simulink model "Local_webcam_test"  (Simulink 7.8)
settings: Solver=ode45  StartTime=0.0  StopTime=10.0  RelTol=1e-3
undefined symbols (not defined in the file): jet, none, videoinput
libraries: visionsinks x2, imaqlib x1
settings Model: Creator=wildcat  LastModifiedBy=wildcat
settings DebuggingCC: FcnCallInpInsideContextMsg=Use local settings  StrictBusMsg=Warning
settings SFSimCC: SimParseCustomCode=off

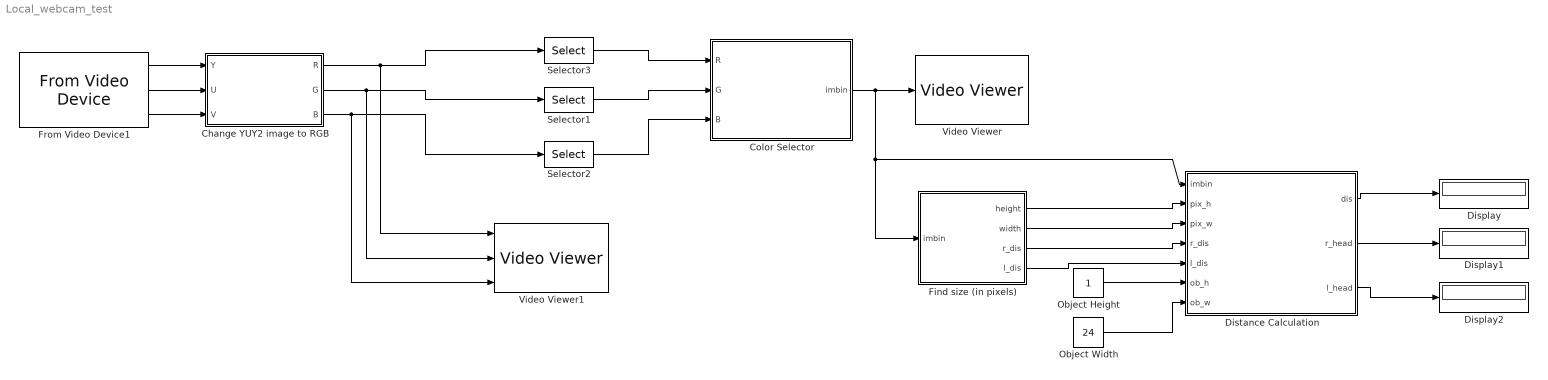
== system Local_webcam_test ==
  Change YUY2 image to RGB : MATLAB Function  TreatAsAtomicUnit=on
  Color Selector : MATLAB Function  TreatAsAtomicUnit=on
  Display : Display
  Display1 : Display
  Display2 : Display
  Distance Calculation : MATLAB Function  TreatAsAtomicUnit=on
  Find size (in pixels) : MATLAB Function  TreatAsAtomicUnit=on
  From Video Device1 : imaqlib/From Video Device  DeviceMenu=winvideo 1 (Microsoft LifeCam HD-3000)  Device=winvideo 1 (Microsoft LifeCam HD-3000)  ObjConstructor=videoinput('winvideo', 1)  VideoFormatMenu=YUY2_640x480  VideoFormat=YUY2_640x480  VideoSource=input1  ROIPosition=[0 0 480 640]  EnableHWTrigger=off  TriggerConfiguration=none/none  SampleTime=1/30  OutputPortsMode=Separate color signals  DataType=uint8  CanDoHWTrigger=no  ReturnedColorSpace=YCbCr  BlockHandle=2599.0059  ROIWidth=640  ROIHeight=480  ROIColumn=0  ROIRow=0  EngXMLPath=C:\Program Files\MatlabR2011b\toolbox\imaq\imaq\private  DevXMLPath=C:\Program Files\MatlabR2011b\toolbox\imaq\imaqadaptors\win64  EngLibPath=C:\Program Files\MatlabR2011b\toolbox\imaq\imaqblks\imaqmex\win64
  Object Height : Constant
  Object Width : Constant  Value=24
  Selector1 : Selector  NumberOfDimensions=2  InputPortWidth=3  IndexOptions=Starting index (dialog),Starting index (dialog)  Indices=70,1  OutputSizes=340,640
  Selector2 : Selector  NumberOfDimensions=2  InputPortWidth=3  IndexOptions=Starting index (dialog),Starting index (dialog)  Indices=70,1  OutputSizes=340,640
  Selector3 : Selector  NumberOfDimensions=2  InputPortWidth=3  IndexOptions=Starting index (dialog),Starting index (dialog)  Indices=70,1  OutputSizes=340,640
  Video Viewer : visionsinks/Video Viewer  inputType=Obsolete7b  imagePorts=One multidimensional signal  useColorMap=off  colormapValue=jet(256)  specRange=off  minInputVal=0  maxInputVal=255  FigPos=[840 554 410 300]  AxisZoom=on  trueSizedOnce=off  OpenAtMdlStart=on
  Video Viewer1 : visionsinks/Video Viewer  inputType=Obsolete7b  imagePorts=Separate color signals  useColorMap=off  colormapValue=jet(256)  specRange=off  minInputVal=0  maxInputVal=255  FigPos=[314 546 410 300]  AxisZoom=on  trueSizedOnce=off  OpenAtMdlStart=on
  wires:
  Color Selector/1(imbin) -> Find size (in pixels)/1(imbin), Distance Calculation/1(imbin), Video Viewer/1
  Find size (in pixels)/1(height) -> Distance Calculation/2(pix_h)
  Find size (in pixels)/2(width) -> Distance Calculation/3(pix_w)
  Object Height/1 -> Distance Calculation/6(ob_h)
  Object Width/1 -> Distance Calculation/7(ob_w)
  Selector3/1 -> Color Selector/1(R)
  Selector1/1 -> Color Selector/2(G)
  Selector2/1 -> Color Selector/3(B)
  Distance Calculation/1(dis) -> Display/1
  Distance Calculation/2(r_head) -> Display1/1
  Distance Calculation/3(l_head) -> Display2/1
  From Video Device1/2 -> Change YUY2 image to RGB/2(U)
  From Video Device1/1 -> Change YUY2 image to RGB/1(Y)
  Change YUY2 image to RGB/1(R) -> Selector3/1, Video Viewer1/1
  Change YUY2 image to RGB/2(G) -> Selector1/1, Video Viewer1/2
  Change YUY2 image to RGB/3(B) -> Selector2/1, Video Viewer1/3
  From Video Device1/3 -> Change YUY2 image to RGB/3(V)
  Find size (in pixels)/3(r_dis) -> Distance Calculation/4(r_dis)
  Find size (in pixels)/4(l_dis) -> Distance Calculation/5(l_dis)

== matlab function Change YUY2 image to RGB ==
  data: Y input double; R output double; G output double; B output double; U input double; V input double
function [R,G,B] = YUY2toRGB(Y,U,V)
%% input is (:,:,1:3), where
%% (:,:,1) is Y, (:,:,2) is U, (:,:,3) is V


%Y = single(data(:,:,1));
%U = single(data(:,:,2));
%V = single(data(:,:,3));

B = 1.164*(Y - 16) + 2.018*(U - 128);

G = 1.164*(Y - 16) - 0.813*(V - 128) - 0.391*(U - 128);

R = 1.164*(Y - 16) + 1.596*(V - 128);

R=uint8(R);
G=uint8(G);
B=uint8(B);

== matlab function Color Selector ==
  data: R input double; G input double; B input double; imbin output double
function imbin  = color_selection(R,G,B)

imsize = size(R);
imsize = size(G);
imsize = size(B);

R1 = zeros(imsize);
G1 = zeros(imsize);
B1 = zeros(imsize);
imbin = zeros(imsize);

for (imh = 1:imsize(1,1));
    for (iml = 1:imsize(1,2));
        imR = R(imh,iml);
        imG = G(imh,iml);
        imB = B(imh,iml);
        if (imR >= 170) && (imR <= 255) && (imG >= 15) && (imG <= 70) && (imB >= 70) && (imB <= 130)
            R1(imh,iml) = 255;
            G1(imh,iml) = 255;
            B1(imh,iml) = 255;
            imbin(imh,iml) = 1;
        end
    end
end

== matlab function Find size (in pixels) ==
  data: imbin input double; height output double; width output double; r_dis output double; l_dis output double
function [height,width,r_dis,l_dis] = hw_find(imbin)

imsize=size(imbin);

height = 0;
width = 0;
height_sum = 0;
width_sum = 0;
marker = 0;
obstart = 0;

for (imh = 1:imsize(1,1));
    width_sum = 0;
    for (iml = 1:imsize(1,2));
        imloc = imbin(imh,iml);
        if (imloc == 1)
            width_sum=width_sum+1;
        end
    end
    if (width_sum >= 6)
        height = height+1;
    end
end



for (iml = 1:imsize(1,2));
    height_sum = 0;
    for (imh = 1:imsize(1,1));
        imloc = imbin(imh,iml);
        if (imloc == 1)
            height_sum=height_sum+1;
        end
    end
    if (height_sum >= 6)
        width = width+1;
        if (marker == 0)
            marker = 1;
            obstart = iml;
        end
    end
end

obend = obstart + width;

r_dis = obstart;
l_dis = imsize(1,2) - obend;

== matlab function Distance Calculation ==
  data: imbin input double; pix_h input double; dis output double; pix_w input double; r_dis input double; l_dis input double; ob_h input double; ob_w input double; r_head output double; l_head output double
function [dis,r_head,l_head] = find_dis(imbin,pix_h,pix_w,r_dis,l_dis,ob_h,ob_w)

%1.4=2*tan(44.443*pi/360)*dis*height1/480;
%ob_w=2*tan(57.154*pi/360)*dis*width1/640;

imsize = size(imbin);

dis1 = (ob_h*imsize(1,1))/(2*tan(44.443*pi/360)*pix_h);

dis2 = (ob_w*imsize(1,2))/(2*tan(57.154*pi/360)*pix_w);


r_head = ob_w*r_dis/pix_w;
%r_head = (ob_w*imsize(1,2))/(2*tan(57.153*pi/360)*pix_w)*(pix_w/r_dis);

l_head = ob_w*l_dis/pix_w;
%l_head = (ob_w*imsize(1,2))/(2*tan(57.153*pi/360)*pix_w)*(pix_w/l_dis);


dis=((dis1*0)+(dis2*1))/1;
